simulink library "models2"  (Simulink 6.0)
values from neighbouring files (symbols this model uses):
  width = abs(diff(LTRB(1:2:3)))    [LTRB2Centre.m]
undefined symbols (not defined in the file or in its folder): beta, C, center, coeffs, delG, exponent, i, initialYValues, interact, invcodeData, invDG, knots, m, maxDelay, n, nhi, nk, nlo, numInputSignals, numterms, orderM, paramIndex, poly_order, polycoeff, polyTerms, reorderM, S, s0, s1, sampleTime, target, WendlandNumTerms, Xvalues
libraries: models2 x45, simulink x17
(part 2 of 2)

== system models2/TwoStage/rbfLogisticEval ==
  X : Inport
  Constant2 : Constant  Value=S  VectorParams1D=off
  Constant3 : Constant  Value=B
  Constant4 : Constant  Value=C  VectorParams1D=off
  Logistic : models2/TwoStage/rbfUtils/Logistic
  Math Function4 : Math  Operator=sqrt  SaturateOnIntegerOverflow=on
  Product4 : Product  Multiplication=Matrix(*)  SaturateOnIntegerOverflow=on  InputSameDT=on
  R : models2/TwoStage/rbfUtils/R
  Y : Outport
  J : Outport  Port=2
  wires:
  Math Function4/1 -> Logistic/1
  Constant3/1 -> Product4/2
  R/1 -> Math Function4/1
  Logistic/1 -> J/1, Product4/1
  Product4/1 -> Y/1
  Constant4/1 -> R/2
  X/1 -> R/1
  Constant2/1 -> R/3

== system models2/TwoStage/rbfMqGlobalWidthEval ==
  X : Inport
  Constant2 : Constant  Value=S  VectorParams1D=off
  Constant3 : Constant  Value=B
  Constant4 : Constant  Value=C  VectorParams1D=off
  MqGlobalWidth : models2/TwoStage/rbfUtils/MqGlobalWidth
  Product4 : Product  Multiplication=Matrix(*)  SaturateOnIntegerOverflow=on  InputSameDT=on
  R : models2/TwoStage/rbfUtils/R
  Y : Outport
  J : Outport  Port=2
  wires:
  R/1 -> MqGlobalWidth/1
  Constant2/1 -> R/3, MqGlobalWidth/2
  X/1 -> R/1
  Constant4/1 -> R/2
  Product4/1 -> Y/1
  MqGlobalWidth/1 -> Product4/1, J/1
  Constant3/1 -> Product4/2

== system models2/TwoStage/rbfMultiquadricEval ==
  X : Inport
  Constant2 : Constant  Value=S  VectorParams1D=off
  Constant3 : Constant  Value=B
  Constant4 : Constant  Value=C  VectorParams1D=off
  Multiquadric : models2/TwoStage/rbfUtils/Multiquadric
  Product4 : Product  Multiplication=Matrix(*)  SaturateOnIntegerOverflow=on  InputSameDT=on
  R : models2/TwoStage/rbfUtils/R
  Y : Outport
  J : Outport  Port=2
  wires:
  Constant3/1 -> Product4/2
  Multiquadric/1 -> J/1, Product4/1
  Product4/1 -> Y/1
  Constant4/1 -> R/2
  X/1 -> R/1
  Constant2/1 -> R/3
  R/1 -> Multiquadric/1

== system models2/TwoStage/rbfRecmqGlobalWidthEval ==
  X : Inport
  Constant2 : Constant  Value=S  VectorParams1D=off
  Constant3 : Constant  Value=B
  Constant4 : Constant  Value=C  VectorParams1D=off
  Math Function : Math  Operator=reciprocal  SaturateOnIntegerOverflow=on
  MqGlobalWidth : models2/TwoStage/rbfUtils/MqGlobalWidth
  Product4 : Product  Multiplication=Matrix(*)  SaturateOnIntegerOverflow=on  InputSameDT=on
  R : models2/TwoStage/rbfUtils/R
  Y : Outport
  J : Outport  Port=2
  wires:
  R/1 -> MqGlobalWidth/1
  Constant2/1 -> R/3, MqGlobalWidth/2
  X/1 -> R/1
  Constant4/1 -> R/2
  Constant3/1 -> Product4/2
  MqGlobalWidth/1 -> Math Function/1
  Product4/1 -> Y/1
  Math Function/1 -> Product4/1, J/1

== system models2/TwoStage/rbfRecmultiquadricEval ==
  X : Inport
  Constant2 : Constant  Value=S  VectorParams1D=off
  Constant3 : Constant  Value=B
  Constant4 : Constant  Value=C  VectorParams1D=off
  Math Function : Math  Operator=reciprocal  SaturateOnIntegerOverflow=on
  Multiquadric : models2/TwoStage/rbfUtils/Multiquadric
  Product4 : Product  Multiplication=Matrix(*)  SaturateOnIntegerOverflow=on  InputSameDT=on
  R : models2/TwoStage/rbfUtils/R
  Y : Outport
  J : Outport  Port=2
  wires:
  Math Function/1 -> J/1, Product4/1
  Product4/1 -> Y/1
  Multiquadric/1 -> Math Function/1
  Constant3/1 -> Product4/2
  Constant4/1 -> R/2
  X/1 -> R/1
  Constant2/1 -> R/3
  R/1 -> Multiquadric/1

== system models2/TwoStage/rbfThinplateEval ==
  X : Inport
  Constant1 : Constant  Value=S  VectorParams1D=off
  Constant2 : Constant  Value=C  VectorParams1D=off
  Constant3 : Constant  Value=B
  Product4 : Product  Multiplication=Matrix(*)  SaturateOnIntegerOverflow=on  InputSameDT=on
  R : models2/TwoStage/rbfUtils/R
  ThinPlate : models2/TwoStage/rbfUtils/ThinPlate
  Y : Outport
  J : Outport  Port=2
  wires:
  Constant3/1 -> Product4/2
  ThinPlate/1 -> J/1, Product4/1
  Product4/1 -> Y/1
  Constant2/1 -> R/2
  X/1 -> R/1
  Constant1/1 -> R/3
  R/1 -> ThinPlate/1

== system models2/TwoStage/rbfUtils ==
  Gaussian : Subsystem
  Logistic : Subsystem
  MqGlobalWidth : Subsystem  AncestorBlock=models2/TwoStage/rbfUtils/Multiquadric
  Multiquadric : Subsystem
  R : Subsystem
  R1 : Subsystem
  RecMultiquadric : Subsystem
  ThinPlate : Subsystem
  Tolerance : Subsystem  mask{V=0, T=eps}
      mask prompts: V "Value to compare"; T "Tolerance"
      mask Display: disp('Tol')
  Wendland : Subsystem  mask{NumTerms=}
      mask prompts: NumTerms "Number of Polynomial Terms"
  arxShellEval : Subsystem
  betaModel_x2fx : Subsystem
  normaliser : Subsystem

== system models2/TwoStage/rbfWendlandEval ==
  X : Inport
  Constant13 : Constant  Value=P
  Constant14 : Constant  Value=E
  Constant2 : Constant  Value=S  VectorParams1D=off
  Constant3 : Constant  Value=B
  Constant4 : Constant  Value=C  VectorParams1D=off
  Math Function4 : Math  Operator=sqrt  SaturateOnIntegerOverflow=on
  Product4 : Product  Multiplication=Matrix(*)  SaturateOnIntegerOverflow=on  InputSameDT=on
  R : models2/TwoStage/rbfUtils/R
  Wendland : Subsystem  AncestorBlock=models2/TwoStage/rbfUtils/Wendland  mask{NumTerms=NumTerms}
      mask prompts: NumTerms "Number of Polynomial Terms"
  Y : Outport
  J : Outport  Port=2
  wires:
  Constant14/1 -> Wendland/3(Exponent)
  Product4/1 -> Y/1
  Wendland/1(P) -> J/1, Product4/1
  Constant3/1 -> Product4/2
  Math Function4/1 -> Wendland/1(R/S)
  Constant4/1 -> R/2
  X/1 -> R/1
  Constant2/1 -> R/3
  R/1 -> Math Function4/1
  Constant13/1 -> Wendland/2(PolyTerms)

== system models2/TwoStage/userModEval ==
  X : Inport
  Y : Outport

== system models2/TwoStage/xreg3xSplineEval ==
  X : Inport
  Constant : Constant  Value=coeffs
  S-Function : S-Function  FunctionName=xreg3xSplineEvalSFnV1  Parameters=orderM,reorderM,knots,poly_order,interact  SFunctionModules=xregsimulinkutils
  Y : Outport
  wires:
  X/1 -> S-Function/2
  S-Function/1 -> Y/1
  Constant/1 -> S-Function/1

== system models2/TwoStageJacob/lollimotJacob ==
  X : Inport
  Jin : Inport  Port=2
  Reshape : simulink/Math Operations/Reshape  OutputDimensionality=1-D array  OutputDimensions=[1,1]
  Selector : Selector  Elements=termsout
  Terminator : Terminator
  J : Outport
  wires:
  X/1 -> Terminator/1
  Jin/1 -> Reshape/1
  Reshape/1 -> Selector/1
  Selector/1 -> J/1

== system models2/TwoStageJacob/mvcubicJacob ==
  X : Inport
  Selector : Selector  Elements=termsout  InputPortWidth=numterms
  mvCubicEval : S-Function  FunctionName=mvCubicJacobSFnV1  Parameters=coeffs,orderM,reorderM
      mask Display: disp('mvCubicJacob');
  J : Outport
  wires:
  Selector/1 -> J/1
  mvCubicEval/1 -> Selector/1
  X/1 -> mvCubicEval/1

== system models2/TwoStageJacob/rbfJacob ==
  X : Inport
  Jin : Inport  Port=2
  Terminator : Terminator
  J : Outport
  wires:
  Jin/1 -> J/1
  X/1 -> Terminator/1

== system models2/TwoStageJacob/userModJacob ==
  X : Inport
  J : Outport

== system models2/TwoStageJacob/xreg3xsplineJacob ==
  X : Inport
  Constant : Constant  Value=coeffs
  S-Function : S-Function  FunctionName=xreg3xSplineJacobSFnV1  Parameters=orderM,reorderM,knots,poly_order,interact  SFunctionModules=xregsimulinkutils
  Selector1 : Selector  Elements=termsout  InputPortWidth=numterms
  J : Outport
  wires:
  Constant/1 -> S-Function/1
  S-Function/1 -> Selector1/1
  X/1 -> S-Function/2
  Selector1/1 -> J/1

== system models2/TwoStageJacob/xregcubicJacob ==
  X : Inport
  Constant : Constant  Value=coeffs
  S-Function : S-Function  FunctionName=mvCubicJacobSFnV2  Parameters=orderM, reorderM, interact
  Selector1 : Selector  Elements=termsout  InputPortWidth=numterms
  J : Outport
  wires:
  Constant/1 -> S-Function/1
  S-Function/1 -> Selector1/1
  X/1 -> S-Function/2
  Selector1/1 -> J/1

== system models2/TwoStageJacob/xreglinear_x2fx ==
  x : Inport
  Constant : Constant
  Mux : Mux  Inputs=2
  fx : Outport
  wires:
  x/1 -> Mux/2
  Mux/1 -> fx/1
  Constant/1 -> Mux/1

== system models2/LocalMod/mmfEval/SubSystem ==
  note: This subsystem ensures that the output
      | is NaN for invalid evaluations
  U : Inport
  V : Inport  Port=2
  Gain : Gain  Gain=-1  SaturateOnIntegerOverflow=on
  Math Function : Math  Operator=pow  OutputSignalType=real  SaturateOnIntegerOverflow=on
  Switch : Switch  InputSameDT=on
  U^V : Outport
  wires:
  Math Function/1 -> U^V/1
  Switch/1 -> Math Function/1
  V/1 -> Math Function/2
  Gain/1 -> Switch/3
  U/1 -> Gain/1, Switch/2, Switch/1

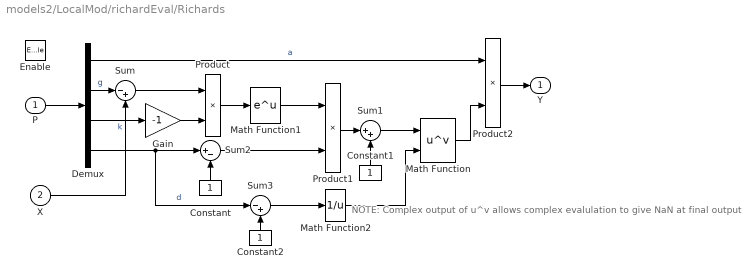
== system models2/LocalMod/richardEval/Richards ==
  note: NOTE: Complex output of u^v allows
      | complex evalulation to give NaN at final output
  P : Inport
  X : Inport  Port=2
  Enable : EnablePort
  Constant : Constant  Orientation=up
  Constant1 : Constant  Orientation=up
  Constant2 : Constant  Orientation=up
  Demux : Demux
  Gain : Gain  Gain=-1  SaturateOnIntegerOverflow=on
  Math Function : Math  Operator=pow  OutputSignalType=complex  SaturateOnIntegerOverflow=on
  Math Function1 : Math  SaturateOnIntegerOverflow=on
  Math Function2 : Math  Operator=reciprocal  SaturateOnIntegerOverflow=on
  Product : Product  SaturateOnIntegerOverflow=on  InputSameDT=on
  Product1 : Product  SaturateOnIntegerOverflow=on  InputSameDT=on
  Product2 : Product  SaturateOnIntegerOverflow=on  InputSameDT=on
  Sum : Sum  Inputs=|-+  SaturateOnIntegerOverflow=on  InputSameDT=on
  Sum1 : Sum  Inputs=|++  SaturateOnIntegerOverflow=on  InputSameDT=on
  Sum2 : Sum  Inputs=|+-  SaturateOnIntegerOverflow=on  InputSameDT=on
  Sum3 : Sum  Inputs=|-+  SaturateOnIntegerOverflow=on  InputSameDT=on
  Y : Outport
  wires:
  P/1 -> Demux/1
  Demux/2 -> Sum/1  "g"
  X/1 -> Sum/2
  Demux/3 -> Gain/1  "k"
  Gain/1 -> Product/2
  Sum/1 -> Product/1
  Product/1 -> Math Function1/1
  Constant/1 -> Sum2/2
  Math Function1/1 -> Product1/1
  Sum2/1 -> Product1/2
  Product1/1 -> Sum1/1
  Constant1/1 -> Sum1/2
  Demux/4 -> Sum3/1, Sum2/1  "d"
  Constant2/1 -> Sum3/2
  Sum3/1 -> Math Function2/1
  Sum1/1 -> Math Function/1
  Math Function2/1 -> Math Function/2
  Demux/1 -> Product2/1  "a"
  Product2/1 -> Y/1
  Math Function/1 -> Product2/2

== system models2/LocalMod/richardEval/Richards  at d == 1 ==
  note: NOTE: Complex output of exp allows
      | complex evalulation of u^v in Richards d~=1
      | to give NaN at final output
  P : Inport
  X : Inport  Port=2
  Enable : EnablePort
  Demux : Demux
  Gain : Gain  Gain=-1  SaturateOnIntegerOverflow=on
  Gain1 : Gain  Gain=-1  SaturateOnIntegerOverflow=on
  Math Function1 : Math  SaturateOnIntegerOverflow=on
  Math Function3 : Math  OutputSignalType=complex  SaturateOnIntegerOverflow=on
  Product : Product  SaturateOnIntegerOverflow=on  InputSameDT=on
  Product2 : Product  SaturateOnIntegerOverflow=on  InputSameDT=on
  Sum : Sum  Inputs=|-+  SaturateOnIntegerOverflow=on  InputSameDT=on
  Terminator : Terminator
  Y : Outport
  wires:
  Demux/4 -> Terminator/1  "d"
  Product2/1 -> Y/1
  Demux/1 -> Product2/1  "a"
  Math Function3/1 -> Product2/2
  Gain1/1 -> Math Function3/1
  Math Function1/1 -> Gain1/1
  Product/1 -> Math Function1/1
  Sum/1 -> Product/1
  Gain/1 -> Product/2
  Demux/3 -> Gain/1  "k"
  X/1 -> Sum/2
  Demux/2 -> Sum/1  "g"
  P/1 -> Demux/1

== system models2/LocalMod/weibulEval/SubSystem ==
  U : Inport
  V : Inport  Port=2
  Gain : Gain  Gain=-1  SaturateOnIntegerOverflow=on
  Gain1 : Gain  Gain=-1  SaturateOnIntegerOverflow=on
  Math Function : Math  Operator=pow  OutputSignalType=real  SaturateOnIntegerOverflow=on
  Math Function1 : Math  SaturateOnIntegerOverflow=on
  Switch : Switch  InputSameDT=on
  e^-(U^V) : Outport
  wires:
  Math Function1/1 -> e^-(U^V)/1
  Math Function/1 -> Gain1/1
  Gain1/1 -> Math Function1/1
  Switch/1 -> Math Function/1
  V/1 -> Math Function/2
  Gain/1 -> Switch/3
  U/1 -> Gain/1, Switch/2, Switch/1

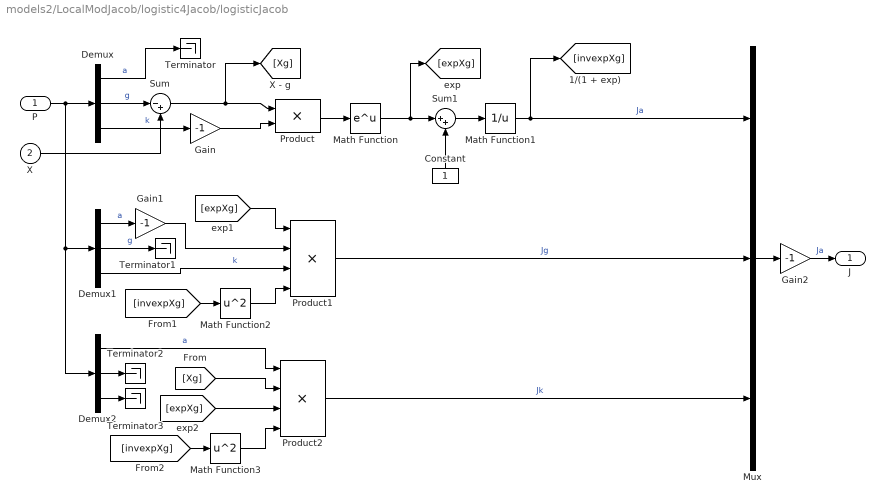
== system models2/LocalModJacob/logistic4Jacob/logisticJacob ==
  P : Inport
  X : Inport  Port=2
  Constant : Constant  Orientation=up
  Demux : Demux  Outputs=3
  Demux1 : Demux  Outputs=3
  Demux2 : Demux  Outputs=3
  Gain : Gain  Gain=-1  SaturateOnIntegerOverflow=on
  Gain1 : Gain  Gain=-1  SaturateOnIntegerOverflow=on
  Gain2 : Gain  Gain=-1  SaturateOnIntegerOverflow=on
  Math Function : Math  SaturateOnIntegerOverflow=on
  Math Function1 : Math  Operator=reciprocal  OutputSignalType=real  SaturateOnIntegerOverflow=on
  Math Function2 : Math  Operator=square  SaturateOnIntegerOverflow=on
  Math Function3 : Math  Operator=square  SaturateOnIntegerOverflow=on
  Mux : Mux  Inputs=3
  Product : Product  SaturateOnIntegerOverflow=on  InputSameDT=on
  Product1 : Product  Inputs=4  SaturateOnIntegerOverflow=on  InputSameDT=on
  Product2 : Product  Inputs=4  SaturateOnIntegerOverflow=on  InputSameDT=on
  Sum : Sum  Inputs=|-+  SaturateOnIntegerOverflow=on  InputSameDT=on
  Sum1 : Sum  Inputs=|++  SaturateOnIntegerOverflow=on  InputSameDT=on
  Terminator{,1..3} (4 alike) : Terminator
  J : Outport
  wires:
  Math Function3/1 -> Product2/4
  [expXg] -> Product2/3
  Product2/1 -> Mux/3  "Jk"
  [Xg] -> Product2/2
  [invexpXg] -> Math Function3/1
  Demux2/1 -> Product2/1  "a"
  Demux2/3 -> Terminator3/1
  Demux2/2 -> Terminator2/1
  Demux1/3 -> Product1/3  "k"
  Product1/1 -> Mux/2  "Jg"
  Math Function2/1 -> Product1/4
  Math Function1/1 -> Mux/1, [invexpXg]  "Ja"
  [invexpXg] -> Math Function2/1
  [expXg] -> Product1/1
  Demux1/2 -> Terminator1/1  "g"
  Gain1/1 -> Product1/2
  Demux1/1 -> Gain1/1  "a"
  Sum1/1 -> Math Function1/1
  Constant/1 -> Sum1/2
  Math Function/1 -> Sum1/1, [expXg]
  Product/1 -> Math Function/1
  Gain/1 -> Product/2
  Demux/3 -> Gain/1  "k"
  Sum/1 -> [Xg], Product/1
  X/1 -> Sum/2
  Demux/2 -> Sum/1  "g"
  Demux/1 -> Terminator/1  "a"
  P/1 -> Demux2/1, Demux1/1, Demux/1
  Mux/1 -> Gain2/1
  Gain2/1 -> J/1  "Ja"

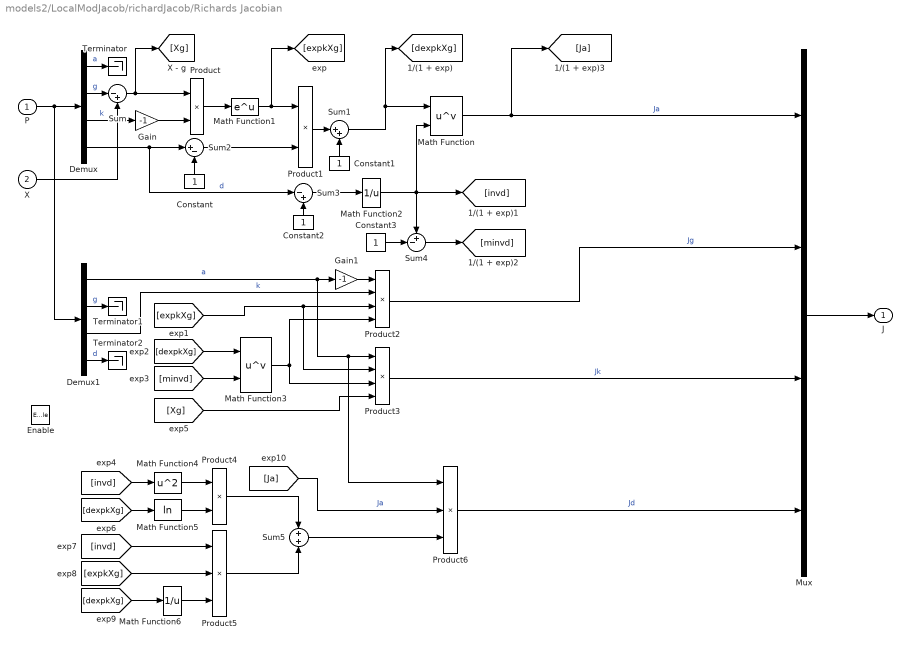
== system models2/LocalModJacob/richardJacob/Richards Jacobian ==
  P : Inport
  X : Inport  Port=2
  Enable : EnablePort
  Constant : Constant  Orientation=up
  Constant1 : Constant  Orientation=up
  Constant2 : Constant  Orientation=up
  Constant3 : Constant
  Demux : Demux
  Demux1 : Demux
  Gain : Gain  Gain=-1  SaturateOnIntegerOverflow=on
  Gain1 : Gain  Gain=-1  SaturateOnIntegerOverflow=on
  Math Function : Math  Operator=pow  SaturateOnIntegerOverflow=on
  Math Function1 : Math  SaturateOnIntegerOverflow=on
  Math Function2 : Math  Operator=reciprocal  SaturateOnIntegerOverflow=on
  Math Function3 : Math  Operator=pow  SaturateOnIntegerOverflow=on
  Math Function4 : Math  Operator=square  SaturateOnIntegerOverflow=on
  Math Function5 : Math  Operator=log  SaturateOnIntegerOverflow=on
  Math Function6 : Math  Operator=reciprocal  SaturateOnIntegerOverflow=on
  Mux : Mux
  Product : Product  SaturateOnIntegerOverflow=on  InputSameDT=on
  Product1 : Product  SaturateOnIntegerOverflow=on  InputSameDT=on
  Product2 : Product  Inputs=4  SaturateOnIntegerOverflow=on  InputSameDT=on
  Product3 : Product  Inputs=4  SaturateOnIntegerOverflow=on  InputSameDT=on
  Product4 : Product  SaturateOnIntegerOverflow=on  InputSameDT=on
  Product5 : Product  Inputs=3  SaturateOnIntegerOverflow=on  InputSameDT=on
  Product6 : Product  Inputs=3  SaturateOnIntegerOverflow=on  InputSameDT=on
  Sum : Sum  Inputs=|-+  SaturateOnIntegerOverflow=on  InputSameDT=on
  Sum1 : Sum  Inputs=|++  SaturateOnIntegerOverflow=on  InputSameDT=on
  Sum2 : Sum  Inputs=|+-  SaturateOnIntegerOverflow=on  InputSameDT=on
  Sum3 : Sum  Inputs=|-+  SaturateOnIntegerOverflow=on  InputSameDT=on
  Sum4 : Sum  Inputs=+-|  SaturateOnIntegerOverflow=on  InputSameDT=on
  Sum5 : Sum  Inputs=+|+  SaturateOnIntegerOverflow=on  InputSameDT=on
  Terminator : Terminator
  Terminator1 : Terminator
  Terminator2 : Terminator
  J : Outport
  wires:
  Demux/2 -> Sum/1  "g"
  X/1 -> Sum/2
  Demux/3 -> Gain/1  "k"
  Product/1 -> Math Function1/1
  Constant/1 -> Sum2/2
  Sum2/1 -> Product1/2
  Product1/1 -> Sum1/1
  Constant1/1 -> Sum1/2
  Sum/1 -> Product/1, [Xg]
  Math Function1/1 -> Product1/1, [expkXg]
  Demux/1 -> Terminator/1  "a"
  Constant2/1 -> Sum3/2
  Sum3/1 -> Math Function2/1
  Demux/4 -> Sum2/1, Sum3/1  "d"
  Sum1/1 -> [dexpkXg], Math Function/1
  Math Function2/1 -> Math Function/2, [invd], Sum4/1
  P/1 -> Demux/1, Demux1/1
  Demux1/2 -> Terminator1/1  "g"
  Demux1/3 -> Product2/2  "k"
  Demux1/4 -> Terminator2/1  "d"
  Product2/1 -> Mux/2  "Jg"
  [expkXg] -> Product2/3, Product3/2
  Gain1/1 -> Product2/1
  Demux1/1 -> Gain1/1, Product3/1, Product6/1  "a"
  Math Function/1 -> [Ja], Mux/1  "Ja"
  [dexpkXg] -> Math Function3/1
  [minvd] -> Math Function3/2
  Math Function3/1 -> Product2/4, Product3/3
  [Xg] -> Product3/4
  Product3/1 -> Mux/3  "Jk"
  [invd] -> Math Function4/1
  [dexpkXg] -> Math Function5/1
  Math Function4/1 -> Product4/1
  Math Function5/1 -> Product4/2
  [expkXg] -> Product5/2
  [invd] -> Product5/1
  Product4/1 -> Sum5/1
  Product5/1 -> Sum5/2
  [Ja] -> Product6/2  "Ja"
  Sum5/1 -> Product6/3
  Product6/1 -> Mux/4  "Jd"
  Gain/1 -> Product/2
  Mux/1 -> J/1
  [dexpkXg] -> Math Function6/1
  Math Function6/1 -> Product5/3
  Sum4/1 -> [minvd]
  Constant3/1 -> Sum4/2

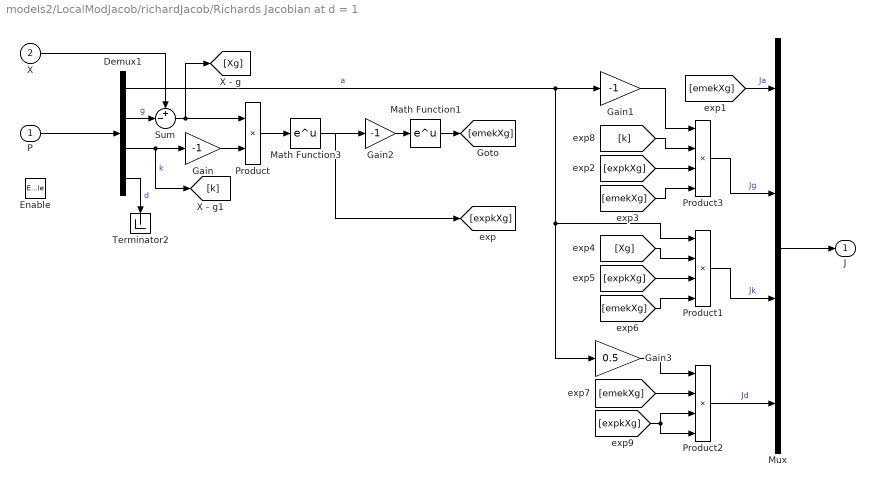
== system models2/LocalModJacob/richardJacob/Richards Jacobian at d = 1 ==
  P : Inport
  X : Inport  Port=2
  Enable : EnablePort
  Demux1 : Demux
  Gain : Gain  Gain=-1  SaturateOnIntegerOverflow=on
  Gain1 : Gain  Gain=-1  SaturateOnIntegerOverflow=on
  Gain2 : Gain  Gain=-1  SaturateOnIntegerOverflow=on
  Gain3 : Gain  Gain=0.5  SaturateOnIntegerOverflow=on
  Math Function1 : Math  SaturateOnIntegerOverflow=on
  Math Function3 : Math  SaturateOnIntegerOverflow=on
  Mux : Mux
  Product : Product  SaturateOnIntegerOverflow=on  InputSameDT=on
  Product1 : Product  Inputs=4  SaturateOnIntegerOverflow=on  InputSameDT=on
  Product2 : Product  Inputs=4  SaturateOnIntegerOverflow=on  InputSameDT=on
  Product3 : Product  Inputs=4  SaturateOnIntegerOverflow=on  InputSameDT=on
  Sum : Sum  Inputs=+-|  SaturateOnIntegerOverflow=on  InputSameDT=on
  Terminator2 : Terminator
      settings: Orientation=down
  J : Outport
  wires:
  P/1 -> Demux1/1
  Gain2/1 -> Math Function1/1
  Math Function1/1 -> [emekXg]
  Mux/1 -> J/1
  [emekXg] -> Mux/1  "Ja"
  Product3/1 -> Mux/2  "Jg"
  Gain1/1 -> Product3/1
  [expkXg] -> Product3/3
  [emekXg] -> Product3/4
  Product1/1 -> Mux/3  "Jk"
  [Xg] -> Product1/2
  [expkXg] -> Product1/3
  [emekXg] -> Product1/4
  Gain3/1 -> Product2/1
  [emekXg] -> Product2/2
  [expkXg] -> Product2/3, Product2/4
  Product2/1 -> Mux/4  "Jd"
  Demux1/3 -> Gain/1, [k]  "k"
  Product/1 -> Math Function3/1
  Sum/1 -> Product/1, [Xg]
  Math Function3/1 -> [expkXg], Gain2/1
  Demux1/1 -> Gain1/1, Product1/1, Gain3/1  "a"
  Gain/1 -> Product/2
  Demux1/4 -> Terminator2/1  "d"
  Demux1/2 -> Sum/2  "g"
  X/1 -> Sum/1
  [k] -> Product3/2

== system models2/LocalModJacob/richardJacob/SubSystem ==
  note: In
  I : Inport
  Abs : Abs  SaturateOnIntegerOverflow=on
  Constant : Constant  Value=V
  Constant1 : Constant  Value=T
  Relational Operator : RelationalOperator  Operator=<=  InputSameDT=on
  Sum : Sum  Inputs=+|-  SaturateOnIntegerOverflow=on  InputSameDT=on
  Out : Outport
  wires:
  Relational Operator/1 -> Out/1
  Constant1/1 -> Relational Operator/2
  Abs/1 -> Relational Operator/1
  Sum/1 -> Abs/1
  Constant/1 -> Sum/2
  I/1 -> Sum/1

== system models2/Reconstruct/gompRecon/Nonlinear reconstruct ==
  P : Inport
  Demux : Demux  Outputs=2
  Gain : Gain  Gain=exp(1)  SaturateOnIntegerOverflow=on
  Product1 : Product  Inputs=/*  SaturateOnIntegerOverflow=on  InputSameDT=on
  k : Outport
  wires:
  P/1 -> Demux/1
  Product1/1 -> k/1
  Demux/1 -> Product1/1  "P"
  Demux/2 -> Gain/1  "Yrf"
  Gain/1 -> Product1/2

== system models2/Reconstruct/localBSplineRecon/Code ==
  K : Inport
  Coded K : Outport

== system models2/Reconstruct/localBSplineRecon/PhiCalc ==
  knots : Inport
  X : Inport  Port=2
  Math Function : Math  Operator=transpose  SaturateOnIntegerOverflow=on
  Reshape : simulink/Math Operations/Reshape  OutputDimensionality=Customize  OutputDimensions=[length(paramIndex), length(paramIndex)]
  S-Function : S-Function  FunctionName=LocalBSplineReconstructSFnV1  Parameters="length(knots),  paramIndex, polyOrder, target"  SFunctionModules=xregsimulinkutils
  delG : Outport
  wires:
  knots/1 -> S-Function/1
  S-Function/1 -> Reshape/1
  X/1 -> S-Function/2
  Reshape/1 -> Math Function/1
  Math Function/1 -> delG/1

== system models2/Reconstruct/localtruncpsRecon/Code ==
  K : Inport
  Coded K : Outport

== system models2/Reconstruct/localtruncpsRecon/fill dG ==
  knots : Inport
  Reshape : simulink/Math Operations/Reshape  OutputDimensionality=Customize  OutputDimensions=size(delG)
  S-Function : S-Function  FunctionName=LocalTruncpsReconstructSFnV1  Parameters=delG, funIndex, polyOrder, Xvalues, derivativeOrder
  delG : Outport
  wires:
  knots/1 -> S-Function/1
  S-Function/1 -> Reshape/1
  Reshape/1 -> delG/1

== system models2/Reconstruct/log4Recon/Nonlinear (Kappa)  reconstruct ==
  note: p(:,4)= Yrf(:,f) + log( (1+p(:,3))./(p(:,3)-1) ) ./p(:,3)
  note: P3
  note: Yrf
  P : Inport
  Constant : Constant
  Constant1 : Constant  Value=1+16*eps
  Demux : Demux  Outputs=2
  Math Function : Math  Operator=log  SaturateOnIntegerOverflow=on
  MinMax : MinMax  Function=max  Inputs=2  SaturateOnIntegerOverflow=on  InputSameDT=on
  Mux : Mux  Inputs=2
  Product : Product  Inputs=/*  SaturateOnIntegerOverflow=on  InputSameDT=on
  Product1 : Product  Inputs=*/  SaturateOnIntegerOverflow=on  InputSameDT=on
  Sum : Sum  Inputs=|+-  SaturateOnIntegerOverflow=on  InputSameDT=on
  Sum1 : Sum  Inputs=++|  SaturateOnIntegerOverflow=on  InputSameDT=on
  Sum2 : Sum  Inputs=+|+  SaturateOnIntegerOverflow=on  InputSameDT=on
  K : Outport
  wires:
  P/1 -> Demux/1
  Constant/1 -> Sum/2, Sum1/1
  Sum/1 -> Product/1
  Sum1/1 -> Product/2
  Product/1 -> Math Function/1
  Math Function/1 -> Product1/1
  Product1/1 -> Sum2/1
  Demux/2 -> Sum2/2
  MinMax/1 -> Sum/1, Sum1/2, Product1/2, Mux/1
  Demux/1 -> MinMax/2
  Constant1/1 -> MinMax/1
  Sum2/1 -> Mux/2
  Mux/1 -> K/1

== system models2/Reconstruct/logRecon/Nonlinear  reconstruct ==
  P : Inport
  Demux : Demux  Outputs=2
  Gain : Gain  Gain=4  SaturateOnIntegerOverflow=on
  Product1 : Product  Inputs=/*  SaturateOnIntegerOverflow=on  InputSameDT=on
  k : Outport
  wires:
  P/1 -> Demux/1
  Product1/1 -> k/1
  Demux/1 -> Product1/1  "P"
  Demux/2 -> Gain/1  "Yrf"
  Gain/1 -> Product1/2

== system models2/Reconstruct/mmfRecon/Nonlinear  reconstruct ==
  P : Inport
  Constant : Constant
  Gain : Gain  Gain=2  SaturateOnIntegerOverflow=on
  Math Function : Math  Operator=reciprocal  SaturateOnIntegerOverflow=on
  Sum : Sum  Inputs=+-|  SaturateOnIntegerOverflow=on  InputSameDT=on
  d : Outport
  wires:
  Math Function/1 -> d/1
  Sum/1 -> Math Function/1
  Constant/1 -> Sum/1
  Gain/1 -> Sum/2
  P/1 -> Gain/1

== system models2/Reconstruct/richReconDelta/Nonlinear  reconstruct ==
  note: p3
  note: p(:,4)= p(:,3)./(2*Yrf(:,f))-1;
      | unless
      | Yrf(:,f) = 0 or p(:,4) = 1
      | then
      | NaN
  P : Inport
  Constant : Constant  Orientation=up
  Constant5 : Constant  Value=NaN
  Demux : Demux  Outputs=2
  Gain : Gain  Gain=2  SaturateOnIntegerOverflow=on
  Hit  Crossing1 : HitCross  HitCrossingOffset=1
  Hit  Crossing2 : HitCross
  Logical Operator : Logic  Operator=OR
  Product : Product  Inputs=*/  SaturateOnIntegerOverflow=on  InputSameDT=on
  Sum : Sum  Inputs=|+-  SaturateOnIntegerOverflow=on  InputSameDT=on
  Switch : Switch  Threshold=0.5  InputSameDT=on
  d : Outport
  wires:
  P/1 -> Demux/1
  Demux/1 -> Product/1
  Gain/1 -> Product/2
  Product/1 -> Sum/1
  Constant/1 -> Sum/2
  Switch/1 -> d/1
  Constant5/1 -> Switch/1
  Logical Operator/1 -> Switch/2
  Hit  Crossing1/1 -> Logical Operator/2
  Hit  Crossing2/1 -> Logical Operator/1
  Sum/1 -> Switch/3, Hit  Crossing1/1
  Demux/2 -> Gain/1, Hit  Crossing2/1  "Yrf"

== system models2/Reconstruct/richReconKappa/Nonlinear  reconstruct ==
  note: p(:,3)= 2*Yrf(:,f)*(p(:,4) + 1);
  note: P4
  P : Inport
  Constant : Constant  Orientation=down
  Demux : Demux  Outputs=2
  Gain : Gain  Gain=2  SaturateOnIntegerOverflow=on
  Product : Product  Inputs=**  SaturateOnIntegerOverflow=on  InputSameDT=on
  Sum1 : Sum  Inputs=++|  SaturateOnIntegerOverflow=on  InputSameDT=on
  d : Outport
  wires:
  Demux/2 -> Gain/1  "Yrf"
  Product/1 -> d/1
  Gain/1 -> Product/2
  P/1 -> Demux/1
  Sum1/1 -> Product/1
  Demux/1 -> Sum1/2
  Constant/1 -> Sum1/1

== system models2/Reconstruct/userLocalRecon/Nonlinear  reconstruct ==
  linP : Inport
  rf : Inport  Port=2
  p : Outport

== system models2/Reconstruct/weibRecon/Nonlinear  reconstruct ==
  note: p(:,3)= ((p(:,4)-1)./p(:,4)).^(1./p(:,4))./Yrf(:,f);
  P1 : Inport
  Constant1 : Constant  Orientation=down
  Demux1 : Demux  Outputs=2
  Math Function2 : Math  Operator=pow  SaturateOnIntegerOverflow=on
  Math Function3 : Math  Operator=reciprocal  SaturateOnIntegerOverflow=on
  Product2 : Product  Inputs=/*  SaturateOnIntegerOverflow=on  InputSameDT=on
  Product3 : Product  Inputs=*/  SaturateOnIntegerOverflow=on  InputSameDT=on
  Sum1 : Sum  Inputs=-+|  SaturateOnIntegerOverflow=on  InputSameDT=on
  d1 : Outport
  wires:
  P1/1 -> Demux1/1
  Constant1/1 -> Sum1/1
  Sum1/1 -> Product2/2
  Demux1/1 -> Sum1/2, Product2/1, Math Function3/1  "P4"
  Product2/1 -> Math Function2/1
  Math Function3/1 -> Math Function2/2
  Math Function2/1 -> Product3/1
  Demux1/2 -> Product3/2  "Yrf"
  Product3/1 -> d1/1

== system models2/TwoStage/rbfUtils/Gaussian ==
  (R/S)^2 : Inport
  Gain1 : Gain  Gain=-1  SaturateOnIntegerOverflow=on
  Math Function2 : Math  SaturateOnIntegerOverflow=on
  P : Outport
  wires:
  Math Function2/1 -> P/1
  (R/S)^2/1 -> Gain1/1
  Gain1/1 -> Math Function2/1  "-(R/S)^2"

== system models2/TwoStage/rbfUtils/Logistic ==
  R/S : Inport
  Constant5 : Constant
  Math Function1 : Math  Operator=reciprocal  SaturateOnIntegerOverflow=on
  Math Function2 : Math  SaturateOnIntegerOverflow=on
  Sum1 : Sum  Inputs=|++  SaturateOnIntegerOverflow=on  InputSameDT=on
  P : Outport
  wires:
  Math Function1/1 -> P/1
  Sum1/1 -> Math Function1/1
  Constant5/1 -> Sum1/2
  Math Function2/1 -> Sum1/1
  R/S/1 -> Math Function2/1

== system models2/TwoStage/rbfUtils/MqGlobalWidth ==
  note: If Sigma has more than one width per dimension
      | then y = sqrt ((R/S)^2 +1)
      | otherwise y = S * sqrt ((R/S)^2 +1)
      |
      | This subsystem deals with the global width case.
      | See Multiquadric for thewidth/dim, width/center
      | and width/center/dim cases.
  (R/S)^2 : Inport
  S : Inport  Port=2
  Constant1 : Constant  Orientation=down
  Math Function2 : Math  Operator=sqrt  SaturateOnIntegerOverflow=on
  Product : Product  SaturateOnIntegerOverflow=on  InputSameDT=on
  Selector : Selector  InputType=Matrix
  Sum : Sum  Inputs=++|  SaturateOnIntegerOverflow=on  InputSameDT=on
  P : Outport
  wires:
  Selector/1 -> Product/2
  Product/1 -> P/1
  Math Function2/1 -> Product/1
  Constant1/1 -> Sum/1
  (R/S)^2/1 -> Sum/2
  Sum/1 -> Math Function2/1
  S/1 -> Selector/1

== system models2/TwoStage/rbfUtils/Multiquadric ==
  note: If Sigma has more than one width per dimension
      | then y = sqrt ((R/S)^2 +1)
      | otherwise y = S * sqrt ((R/S)^2 +1)
      |
      | This subsystem deals with the width/dim, width/center
      | and width/center/dim cases. See MqGlobalWidth
      | for the global width case
  (R/S)^2 : Inport
  Constant1 : Constant  Orientation=down
  Math Function2 : Math  Operator=sqrt  SaturateOnIntegerOverflow=on
  Sum : Sum  Inputs=++|  SaturateOnIntegerOverflow=on  InputSameDT=on
  P : Outport
  wires:
  Sum/1 -> Math Function2/1
  (R/S)^2/1 -> Sum/2
  Constant1/1 -> Sum/1
  Math Function2/1 -> P/1

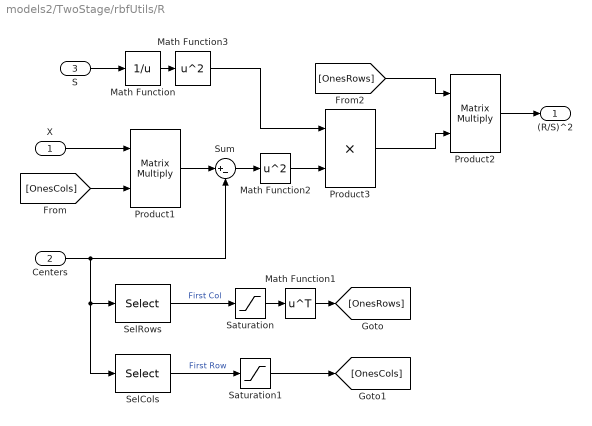
== system models2/TwoStage/rbfUtils/R ==
  X : Inport
  "Centers " : Inport  Port=2
  S : Inport  Port=3
  Math Function : Math  Operator=reciprocal  SaturateOnIntegerOverflow=on
  Math Function1 : Math  Operator=transpose  SaturateOnIntegerOverflow=on
  Math Function2 : Math  Operator=square  SaturateOnIntegerOverflow=on
  Math Function3 : Math  Operator=square  SaturateOnIntegerOverflow=on
  Product1 : Product  Multiplication=Matrix(*)  SaturateOnIntegerOverflow=on  InputSameDT=on
  Product2 : Product  Multiplication=Matrix(*)  SaturateOnIntegerOverflow=on  InputSameDT=on
  Product3 : Product  SaturateOnIntegerOverflow=on  InputSameDT=on
  Saturation : Saturate  UpperLimit=1  LowerLimit=1
  Saturation1 : Saturate  UpperLimit=1  LowerLimit=1
  SelCols : Selector  InputType=Matrix  Elements=[1 3]  Columns=-1  InputPortWidth=3
  SelRows : Selector  InputType=Matrix  Elements=[1 3]  Rows=-1  InputPortWidth=3
  Sum : Sum  Inputs=|+-  SaturateOnIntegerOverflow=on  InputSameDT=on
  (R/S)^2 : Outport
  wires:
  Math Function2/1 -> Product3/2
  Sum/1 -> Math Function2/1
  Product1/1 -> Sum/1
  X/1 -> Product1/1
  [OnesCols] -> Product1/2
  Math Function1/1 -> [OnesRows]
  SelRows/1 -> Saturation/1  "First Col"
  "Centers "/1 -> Sum/2, SelRows/1, SelCols/1
  S/1 -> Math Function/1
  Math Function/1 -> Math Function3/1
  Saturation/1 -> Math Function1/1
  SelCols/1 -> Saturation1/1  "First Row"
  Saturation1/1 -> [OnesCols]
  Math Function3/1 -> Product3/1
  Product3/1 -> Product2/2
  Product2/1 -> (R/S)^2/1
  [OnesRows] -> Product2/1

== system models2/TwoStage/rbfUtils/R1 ==
  X : Inport
  Constant1 : Constant  Value=S  VectorParams1D=off
  Constant2 : Constant  Value=C  VectorParams1D=off
  Math Function : Math  Operator=reciprocal  SaturateOnIntegerOverflow=on
  Math Function2 : Math  Operator=square  SaturateOnIntegerOverflow=on
  Math Function3 : Math  Operator=square  SaturateOnIntegerOverflow=on
  OnesC : Constant  Value=ones(1, size(C, 2))  VectorParams1D=off
  OnesD : Constant  Value=ones(1, size(C, 1))  VectorParams1D=off
  Product1 : Product  Multiplication=Matrix(*)  SaturateOnIntegerOverflow=on  InputSameDT=on
  Product2 : Product  Multiplication=Matrix(*)  SaturateOnIntegerOverflow=on  InputSameDT=on
  Product3 : Product  SaturateOnIntegerOverflow=on  InputSameDT=on
  Sum : Sum  Inputs=|+-  SaturateOnIntegerOverflow=on  InputSameDT=on
  (R/S)^2 : Outport
  wires:
  OnesD/1 -> Product2/1  "1 x nD"
  Product2/1 -> (R/S)^2/1  "1 x nC"
  Product3/1 -> Product2/2  "nD x nC"
  Constant1/1 -> Math Function/1
  Math Function/1 -> Math Function3/1
  Math Function3/1 -> Product3/2  "nD x nC"
  Math Function2/1 -> Product3/1  "nD x nC"
  Sum/1 -> Math Function2/1
  Product1/1 -> Sum/1
  X/1 -> Product1/1  "nD x 1"
  OnesC/1 -> Product1/2  "1 x nC"
  Constant2/1 -> Sum/2  "nD x nC"

== system models2/TwoStage/rbfUtils/RecMultiquadric ==
  note: RecMultiquadric = 1/ sqrt( (R/S)^2 + 1 )
  (R/S)^2 : Inport
  Constant : Constant
  Math Function2 : Math  Operator=sqrt  SaturateOnIntegerOverflow=on
  Math Function3 : Math  Operator=reciprocal  SaturateOnIntegerOverflow=on
  Sum : Sum  Inputs=|++  SaturateOnIntegerOverflow=on  InputSameDT=on
  P : Outport
  wires:
  Math Function3/1 -> P/1
  Math Function2/1 -> Math Function3/1
  (R/S)^2/1 -> Sum/1
  Sum/1 -> Math Function2/1  "(R/S)^2+1"
  Constant/1 -> Sum/2

== system models2/TwoStage/rbfUtils/ThinPlate ==
  (R/S)^2 : Inport
  Constant1 : Constant  Orientation=up  Value=0
  Math Function1 : Math  Operator=sqrt  SaturateOnIntegerOverflow=on
  Math Function2 : Math  Operator=log  SaturateOnIntegerOverflow=on
  Product2 : Product  SaturateOnIntegerOverflow=on  InputSameDT=on
  Switch : Switch  Criteria=u2 ~= 0  InputSameDT=on
  P : Outport
  wires:
  Switch/1 -> P/1
  Product2/1 -> Switch/1
  Constant1/1 -> Switch/3
  Math Function1/1 -> Math Function2/1
  (R/S)^2/1 -> Math Function1/1, Product2/1, Switch/2
  Math Function2/1 -> Product2/2

== system models2/TwoStage/rbfUtils/Tolerance ==
  I : Inport
  Abs : Abs  SaturateOnIntegerOverflow=on
  Constant : Constant  Value=V
  Constant1 : Constant  Value=T
  Relational Operator : RelationalOperator  Operator=<=  InputSameDT=on
  Sum : Sum  Inputs=+|-  SaturateOnIntegerOverflow=on  InputSameDT=on
  Out : Outport
  wires:
  I/1 -> Sum/1
  Constant/1 -> Sum/2
  Sum/1 -> Abs/1
  Abs/1 -> Relational Operator/1
  Constant1/1 -> Relational Operator/2
  Relational Operator/1 -> Out/1

== system models2/TwoStage/rbfUtils/Wendland ==
  R/S : Inport
  PolyTerms : Inport  Port=2
  Exponent : Inport  Port=3
  Constant : Constant
  Constant1 : Constant  Value=0
  Math Function : Math  Operator=pow  SaturateOnIntegerOverflow=on
  Product : Product  SaturateOnIntegerOverflow=on  InputSameDT=on
  S-Function : S-Function  FunctionName=WendlandEvalSFnV1  Parameters=NumTerms
  Sum : Sum  Inputs=-+|  SaturateOnIntegerOverflow=on  InputSameDT=on
  Switch : Switch  InputSameDT=on
  P : Outport
  wires:
  Switch/1 -> Product/2
  Math Function/1 -> Switch/1, Switch/2
  S-Function/1 -> Product/1
  Constant1/1 -> Switch/3
  Exponent/1 -> Math Function/2
  Sum/1 -> Math Function/1
  Constant/1 -> Sum/2
  PolyTerms/1 -> S-Function/1
  R/S/1 -> Sum/1, S-Function/2  "R/S"
  Product/1 -> P/1

== system models2/TwoStage/rbfUtils/arxShellEval ==
  X : Inport
  Initial Value : Subsystem  AncestorBlock=FordExtrasSimulinkModels/TwoStage/rbfUtils/arxShellEval/Initial Value  mask{sampleTime=sampleTime, initialValues=initialYValues}
      mask prompts: sampleTime "Sample Time"; initialValues "Initial Y value"
  InvCode : Subsystem
  JacobInvCode : Subsystem
  Mux : Mux  Inputs=2
  Selector : Selector  Elements=selectedSignals  InputPortWidth=maxDelay*(numInputSignals+1)
  X Delay : Subsystem  mask{numSignals=numInputSignals}
      mask prompts: numSignals "Number of Input Siganls"
  Y Delay : Subsystem
  kernel : Subsystem
  Y : Outport
  J : Outport  Port=2
  wires:
  JacobInvCode/1(J) -> J/1
  InvCode/1(Y) -> Y/1
  Selector/1 -> kernel/1(X)
  X Delay/1(delayed X) -> Mux/1
  X/1 -> X Delay/1(X)
  kernel/1(Y) -> Initial Value/1(Yin)
  Initial Value/1(Y) -> InvCode/1(Y Coded), Y Delay/1(Y)
  Y Delay/1(delayed Y) -> Mux/2
  Mux/1 -> Selector/1
  kernel/2(J) -> JacobInvCode/1(J Coded)

== system models2/TwoStage/rbfUtils/betaModel_x2fx ==
  note: This subsystem is a place to put the X2FX block
      | for the beta models inside a Lolimot model.
  x : Inport
  fx : Outport

== system models2/TwoStage/rbfUtils/normaliser ==
  P : Inport
  Constant : Constant  Orientation=up  Value=ones(1, size(C, 2))
  Constant1 : Constant  Value=eps
  Dot Product : simulink/Math Operations/Dot Product  OutDataType=sfix(16)  OutScaling=2^-10  DoSatur=off
  Product : Product  Inputs=*/  SaturateOnIntegerOverflow=on  InputSameDT=on
  Switch : Switch  Threshold=1  SaturateOnIntegerOverflow=on  InputSameDT=on
  Tolerance : models2/TwoStage/rbfUtils/Tolerance  V=0  T=eps
  normP : Outport
  wires:
  Switch/1 -> Product/2
  Tolerance/1 -> Switch/2
  Product/1 -> normP/1
  Dot Product/1 -> Switch/3, Tolerance/1
  Constant/1 -> Dot Product/2
  P/1 -> Dot Product/1, Product/1
  Constant1/1 -> Switch/1

== system models2/TwoStage/rbfWendlandEval/Wendland ==
  R/S : Inport
  PolyTerms : Inport  Port=2
  Exponent : Inport  Port=3
  Constant : Constant
  Constant1 : Constant  Value=0
  Math Function1 : Math  Operator=pow  SaturateOnIntegerOverflow=on
  Product : Product  SaturateOnIntegerOverflow=on  InputSameDT=on
  S-Function : S-Function  FunctionName=WendlandEvalSFnV1  Parameters=NumTerms
  Sum : Sum  Inputs=-+|  SaturateOnIntegerOverflow=on  InputSameDT=on
  Switch : Switch  InputSameDT=on
  P : Outport
  wires:
  Product/1 -> P/1
  R/S/1 -> S-Function/2, Sum/1  "R/S"
  PolyTerms/1 -> S-Function/1
  Constant/1 -> Sum/2
  Exponent/1 -> Math Function1/2
  Constant1/1 -> Switch/3
  S-Function/1 -> Product/1
  Sum/1 -> Math Function1/1, Switch/2
  Math Function1/1 -> Switch/1
  Switch/1 -> Product/2

== system models2/TwoStage/rbfUtils/arxShellEval/Initial Value ==
  Yin : Inport  Orientation=down
  Count : Subsystem  mask{sampleTime=sampleTime, count=length(initialValues)}
      mask prompts: sampleTime "Sample Time"
  Enabled Subsystem : Subsystem  TreatAsAtomicUnit=on
  Logical Operator : Logic  Orientation=down  Operator=NOT
  Switch : Switch  Threshold=1  SaturateOnIntegerOverflow=on  InputSameDT=on
  Y : Outport
  wires:
  Logical Operator/1 -> Enabled Subsystem/Enable
  Enabled Subsystem/1(initialValue(t)) -> Switch/3
  Count/2(timestep) -> Enabled Subsystem/1(t)
  Yin/1 -> Switch/1
  Switch/1 -> Y/1
  Count/1(count Exceeded) -> Logical Operator/1, Switch/2

== system models2/TwoStage/rbfUtils/arxShellEval/InvCode ==
  Y Coded : Inport
  Constant : Constant  Orientation=up  Value=invcodeData(1)
  Gain : Gain  Gain=invcodeData(2)  SaturateOnIntegerOverflow=on
  Sum : Sum  Inputs=|++  SaturateOnIntegerOverflow=on  InputSameDT=on
  Y : Outport
  wires:
  Y Coded/1 -> Gain/1
  Sum/1 -> Y/1
  Constant/1 -> Sum/2
  Gain/1 -> Sum/1

== system models2/TwoStage/rbfUtils/arxShellEval/JacobInvCode ==
  J Coded : Inport
  Gain : Gain  Gain=invcodeData(2)  SaturateOnIntegerOverflow=on
  J : Outport
  wires:
  Gain/1 -> J/1
  J Coded/1 -> Gain/1

== system models2/TwoStage/rbfUtils/arxShellEval/X Delay ==
  X : Inport
  Matrix Concatenation : simulink/Math Operations/Matrix Concatenation  numInports=2  catMethod=Vertical
  Reshape : simulink/Math Operations/Reshape  OutputDimensionality=Row vector  OutputDimensions=[1,1]
  Reshape1 : simulink/Math Operations/Reshape  Orientation=left  OutputDimensionality=Customize  OutputDimensions=[maxDelay, numSignals]
  Reshape2 : simulink/Math Operations/Reshape  OutputDimensionality=1-D array  OutputDimensions=[1,1]
  Selector : Selector  Orientation=left  InputType=Matrix  Elements=1:4  Rows=1:maxDelay-1  Columns=-1  InputPortWidth=5
  Unit Delay : UnitDelay  Orientation=left  X0=zeros(maxDelay, numSignals)  SampleTime=sampleTime
  Zero-Order Hold : ZeroOrderHold  SampleTime=sampleTime
  delayed X : Outport
  wires:
  Selector/1 -> Matrix Concatenation/2
  Matrix Concatenation/1 -> Unit Delay/1, Reshape2/1
  X/1 -> Zero-Order Hold/1
  Reshape/1 -> Matrix Concatenation/1
  Reshape1/1 -> Selector/1
  Unit Delay/1 -> Reshape1/1
  Zero-Order Hold/1 -> Reshape/1
  Reshape2/1 -> delayed X/1

== system models2/TwoStage/rbfUtils/arxShellEval/Y Delay ==
  Y : Inport
  Constant : Constant  Orientation=down  Value=NaN
  Mux : Mux  Inputs=2
  Mux1 : Mux  Inputs=2
  Selector : Selector  Orientation=left  Elements=1:maxDelay-1  Rows=1:maxDelay-1  Columns=-1  InputPortWidth=maxDelay
  Selector1 : Selector  Elements=1:maxDelay  Rows=1:maxDelay-1  Columns=-1  InputPortWidth=maxDelay+1
  Unit Delay : UnitDelay  SampleTime=sampleTime
  delayed Y : Outport
  wires:
  Y/1 -> Mux/1
  Mux/1 -> Unit Delay/1
  Selector/1 -> Mux/2
  Unit Delay/1 -> Selector/1, Mux1/2
  Constant/1 -> Mux1/1
  Mux1/1 -> Selector1/1
  Selector1/1 -> delayed Y/1

== system models2/TwoStage/rbfUtils/arxShellEval/kernel ==
  X : Inport
  Y : Outport
  J : Outport  Port=2

== system models2/TwoStage/rbfUtils/arxShellEval/Initial Value/Count ==
  Constant : Constant
  Constant1 : Constant  Orientation=up  Value=count
  Relational Operator1 : RelationalOperator  Operator=>  InputSameDT=on
  Sum1 : Sum  Inputs=++|  SaturateOnIntegerOverflow=on  InputSameDT=on
  Unit Delay1 : UnitDelay  Orientation=left  SampleTime=sampleTime
  count Exceeded : Outport
  timestep : Outport  Port=2
  wires:
  Unit Delay1/1 -> Sum1/1
  Relational Operator1/1 -> count Exceeded/1
  Constant/1 -> Sum1/2
  Constant1/1 -> Relational Operator1/2
  Sum1/1 -> timestep/1, Unit Delay1/1, Relational Operator1/1

== system models2/TwoStage/rbfUtils/arxShellEval/Initial Value/Enabled Subsystem ==
  t : Inport
  Enable : EnablePort
  Constant1 : Constant  Value=initialValues
  Selector : Selector  ElementSrc=External  Elements=[1 3]  InputPortWidth=length(initialValues)
  initialValue(t) : Outport
  wires:
  t/1 -> Selector/2
  Selector/1 -> initialValue(t)/1
  Constant1/1 -> Selector/1
